simulink model "Stinger"  (R2023a)
settings: Solver=VariableStepAuto  StartTime=0.0  StopTime=20  FixedStep=1e-3  EnableMultiTasking=on
values from neighbouring files (symbols this model uses):
  bp = 0.001    [ControlLawsScript.m]    (also in ControlLaws_Script.m)
  bq = 0.001    [ControlLawsScript.m]    (also in ControlLaws_Script.m)
  br = 0.001    [ControlLawsScript.m]    (also in ControlLaws_Script.m)
  cx = 5    [ControlLawsScript.m]    (also in ControlLaws_Script.m)
  cy = 5    [ControlLawsScript.m]    (also in ControlLaws_Script.m)
  cz = 5    [ControlLawsScript.m]    (also in ControlLaws_Script.m)
  g = 9.80665    [ControlLawsScript.m]    (also in ControlLaws_Script.m; Qball_X8_Model.m = 9.87)
  Kp = (Jx/Tc)-bp    (= 1.02772632451)    [ControlLawsScript.m]    (also in ControlLaws_Script.m = 4.11390529802)
  Kp2 = Jx*((4/ts))*((-4/ts)+((bp+Kp)/Jx))/Kp    (= 1.68163467643)    [ControlLawsScript.m]    (also in ControlLaws_Script.m = 6.72163348437)
  Kq = (Jy/Tc)-bq    (= 1.02971502036)    [ControlLawsScript.m]    (also in ControlLaws_Script.m = 4.12186008142)
  Kq2 = Jy*((4/ts))*((-4/ts)+((bq+Kq)/Jy))/Kq    (= 1.68163151937)    [ControlLawsScript.m]    (also in ControlLaws_Script.m = 6.72163033191)
  Kr = (Jz/Tc)-br    (= 1.98490876719)    [ControlLawsScript.m]    (also in ControlLaws_Script.m = 7.94263506876)
  Kr2 = Jz*((4/ts))*((-4/ts)+((br+Kr)/Jz))/Kr    (= 1.68084638651)    [ControlLawsScript.m]    (also in ControlLaws_Script.m = 6.72084606682)
  kv = 1/930    (= 0.0010752688172)    [StingerScript.m]
  Kx = abs(Kx)    [ControlLawsScript.m]    (also in ControlLaws_Script.m)
  Ky = abs(Ky)    [ControlLawsScript.m]    (also in ControlLaws_Script.m)
  Kz = (m/Tcz)-cz    (= 38.5143536865)    [ControlLawsScript.m]    (also in ControlLaws_Script.m)
  Kz2 = m*((4/tsz))*((-4/tsz)+((cz+Kz)/m))/Kz    (= 1.89810050529)    [ControlLawsScript.m]    (also in ControlLaws_Script.m)
  m = 3.4811482949175    (= 3.48114829492)    [ControlLawsScript.m]    (also in ControlLaws_Script.m; Qball_X8_Model.m = 1.45)
  pitch_angle_limit = pi/6    (= 0.523598775598)    [ControlLawsScript.m]    (also in ControlLaws_Script.m = 0.558505360638)
  R2D = 180/pi    (= 57.2957795131)    [ControlLawsScript.m]    (also in ControlLaws_Script.m)
  roll_angle_limit = pi/6    (= 0.523598775598)    [ControlLawsScript.m]    (also in ControlLaws_Script.m = 0.558505360638)
  z_x = cx    (= 5)    [ControlLawsScript.m]    (also in ControlLaws_Script.m)
  z_y = cy    (= 5)    [ControlLawsScript.m]    (also in ControlLaws_Script.m)
undefined symbols (not defined in the file or in its folder): FC, LAC, LeftAftArm, LeftAftProp, LeftAftSkid, LeftArm, LeftFrontArm, LeftFrontProp, LeftFrontSkid, LeftProp, Lower, missionPlanX, missionPlanY, missionPlanYaw, missionPlanZ, RAC, RightAftArm, RightAftProp, RightAftSkid, RightArm, RightFrontArm, RightFrontProp, RightFrontSkid, RightProp, SC, timeConstant, Upper, X, Y, Z
libraries: sm_lib x98, nesl_utility x56, fl_lib x45, ee_lib x19, batteryecm_lib x2, sharedtransformsys x1, sharedutil x1
(part 1 of 4)
settings Model: Creator=G_MAMAN  LastModifiedBy=alger
settings SolverCC: ZeroCrossAlgorithm=Adaptive  AlgebraicLoopSolver=LineSearch  SolverResetMethod=Robust
settings DataIOCC: LimitDataPoints=on  MaxDataPoints=10000  Refine=5
settings OptimizationCC: LifeSpan=inf
settings DebuggingCC: IgnoredZcDiagnostic=none  UnconnectedInputMsg=warning  UnconnectedOutputMsg=warning  UnconnectedLineMsg=warning  AllowSymbolicDim=off  SFUnexpectedBacktrackingDiag=warning  SFNoUnconditionalDefaultTransitionDiag=warning  SFExecutionAtInitializationDiag=none  ArithmeticOperatorsInVariantConditions=warning
settings ModelReferenceCC: EnableRefExpFcnMdlSchedulingChecks=on
settings SFSimCC: SimUseLocalCustomCode=off  CustomCodeUndefinedFunction=UseInterfaceOnly
settings RTWCC: RTWUseLocalCustomCode=off
settings CodeAppCC: StateflowObjectComments=on
settings GRTTargetCC: TargetLangStandard=C89/C90 (ANSI)
settings ConfigComp: CovMetricSettings=dw  CovSaveCumulativeToWorkspaceVar=on  CovSaveSingleToWorkspaceVar=on  CovExternalEMLEnable=off  CovSFcnEnable=off
settings SimscapeCC: SimscapeLogType=all  SimscapeLogSimulationStatistics=on  SimscapeLogDataHistory=10000
settings DiagnosticsConfigSet: SimMechanicsRigidlyBoundBlock=none
settings ExplorerConfigSet: InternalSimMechanicsExplorerSettings="<ExplorerConfiguration><canonicalview>default</canonicalview><AnimationSetting><BasePlaybackSpeed>1.0</BasePlaybackSpeed><PlaybackSpeedFactor>1.0</PlaybackSpeedFactor></AnimationSetting><TilePanel><TileInfo><Tiles Columns=\"1\" Count=\"1\" Rows=\"1\"><Column Weight=\"1\"/><Row Weight=\"1\"/><Tile Height=\"1\" Width=\"1\" X=\"0\" Y=\"0\"/></Tiles></TileInfo><SceneInfo><SceneViewer><BGColor><R>0</R><G>0</G><B>0</B></BGColor><Camera><DoPerspective>off</DoPerspective><Position><X>7.1395388580893373</X><Y>-9.57545541238177833</Y><Z>5.80767107239631564</Z></Position><Center><X>-0.863567299281931766</X><Y>0.176174380151177173</Y><Z>1.92916926391305155</Z></Center><Up><X>-0.173509302469238902</X><Y>0.237715937307242831</Y><Z>0.955712119367949198</Z></Up><ViewLimDist>1</ViewLimDist><YLim>4.19925208742349287</YLim><XLim>9.96419089960335391</XLim></Camera></SceneViewer></SceneInfo></TilePanel><MechEditorPanel><Cameras/><GfxPanelCameraMap/><VideoCreator><PlaybackSpeedRatio>1.0</PlaybackSpeedRatio><FrameRate>30</FrameRate><VideoFormat>Motion JPEG AVI</VideoFormat><FrameSize>auto</FrameSize></VideoCreator></MechEditorPanel></ExplorerConfiguration>"

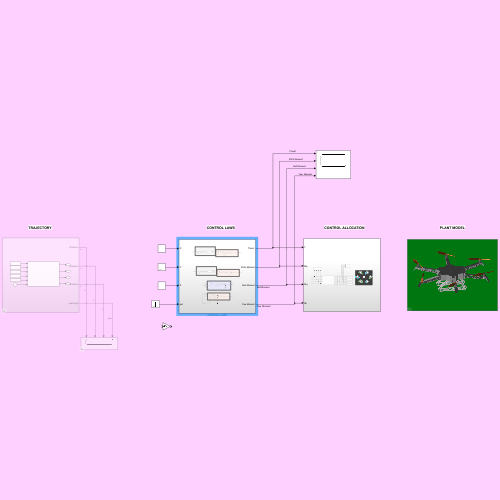
[thumbnail: Simulink's stored preview of the top-level diagram]
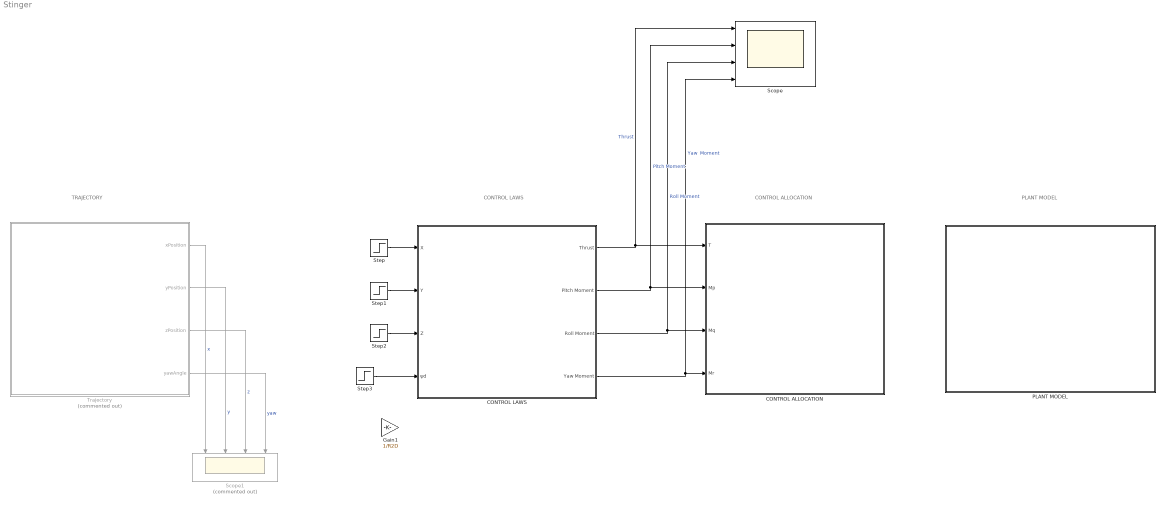
== system Stinger ==
  note: CONTROL LAWS
  note: CONTROL ALLOCATION
  note: PLANT MODEL
  note: TRAJECTORY
  CONTROL ALLOCATION : Subsystem
  CONTROL LAWS : Subsystem
  Gain1 : Gain  Gain=1/R2D
  PLANT MODEL : Subsystem  mask{s=6, g=9.80665, D=0.235, H=0.051, rho=3400, rgb=[0.753 0.753 0.753], op=1}
      mask prompts: s "Shape (# Sides)"; g "Gravitational Acceleration (m/s^2)"; D "Length of Fuselage (m)"; H "Height of Fuselage (m)"; rho "Density of Fuselage (kg/m^3)"; rgb "Color of Fuselage [R G B]"; op "Opacity of Fuselage (0-1)"
      mask Display: image('$imagefile'); % Use "Edit Image" on toolstrip to change.
  Scope : Scope  NumInputPorts=4
  Scope1 : Scope  Commented=on  NumInputPorts=4
  Step : Step  Time=0  After=0  SampleTime=0
  Step1 : Step  Time=0  After=0  SampleTime=0
  Step2 : Step  Time=0  After=4  SampleTime=0
  Step3 : Step  Time=4  After=2  SampleTime=0
  Trajectory : Subsystem  Commented=on
  wires:
  CONTROL LAWS/4(Yaw Moment) -> Scope/4, CONTROL ALLOCATION/4(Mr)  "Yaw  Moment"
  CONTROL LAWS/2(Pitch Moment) -> Scope/2, CONTROL ALLOCATION/2(Mp)  "Pitch Moment"
  CONTROL LAWS/1("Thrust ") -> Scope/1, CONTROL ALLOCATION/1(T)  "Thrust"
  CONTROL LAWS/3(Roll Moment) -> Scope/3, CONTROL ALLOCATION/3(Mq)  "Roll Moment"
  Trajectory/1(xPosition) -> Scope1/1  "x"
  Trajectory/2(yPosition) -> Scope1/2  "y"
  Trajectory/3(zPosition) -> Scope1/3  "z"
  Trajectory/4(yawAngle) -> Scope1/4  "yaw"
  Step/1 -> CONTROL LAWS/1(X)
  Step1/1 -> CONTROL LAWS/2(Y)
  Step2/1 -> CONTROL LAWS/3(Z)
  Step3/1 -> CONTROL LAWS/4(ψd)

== system Stinger/CONTROL ALLOCATION ==
  note: 1
  T : Inport
  Mp : Inport  Port=2
  Mq : Inport  Port=3
  Mr : Inport  Port=4
  Control Allocation : MATLAB Function  TreatAsAtomicUnit=on
  Saturation{6..11} (6 alike) : Saturate  UpperLimit=10000  LowerLimit=0
  Scope : Scope  NumInputPorts=4
  Scope1 : Scope  NumInputPorts=6
  tag scope: ReqSpeedMotor1=global, ReqSpeedMotor2=global, ReqSpeedMotor3=global, ReqSpeedMotor4=global, ReqSpeedMotor5=global, ReqSpeedMotor6=global
  wires:
  T/1 -> Control Allocation/1(T), Scope/1  "T"
  Mp/1 -> Control Allocation/2(Mp), Scope/2  "Mp"
  Mq/1 -> Control Allocation/3(Mq), Scope/3  "Mq"
  Mr/1 -> Control Allocation/4(Mr), Scope/4  "Mr"
  Control Allocation/1(w1) -> Saturation6/1  "1"
  Control Allocation/2(w2) -> Saturation7/1  "2"
  Control Allocation/3(w3) -> Saturation8/1  "3"
  Control Allocation/4(w4) -> Saturation9/1  "4"
  Control Allocation/6(w6) -> Saturation11/1  "6"
  Control Allocation/5(w5) -> Saturation10/1  "5"
  Saturation6/1 -> [ReqSpeedMotor1], Scope1/1
  Saturation10/1 -> Scope1/5, [ReqSpeedMotor5]
  Saturation7/1 -> [ReqSpeedMotor2], Scope1/2
  Saturation9/1 -> Scope1/4, [ReqSpeedMotor4]
  Saturation8/1 -> Scope1/3, [ReqSpeedMotor3]
  Saturation11/1 -> Scope1/6, [ReqSpeedMotor6]

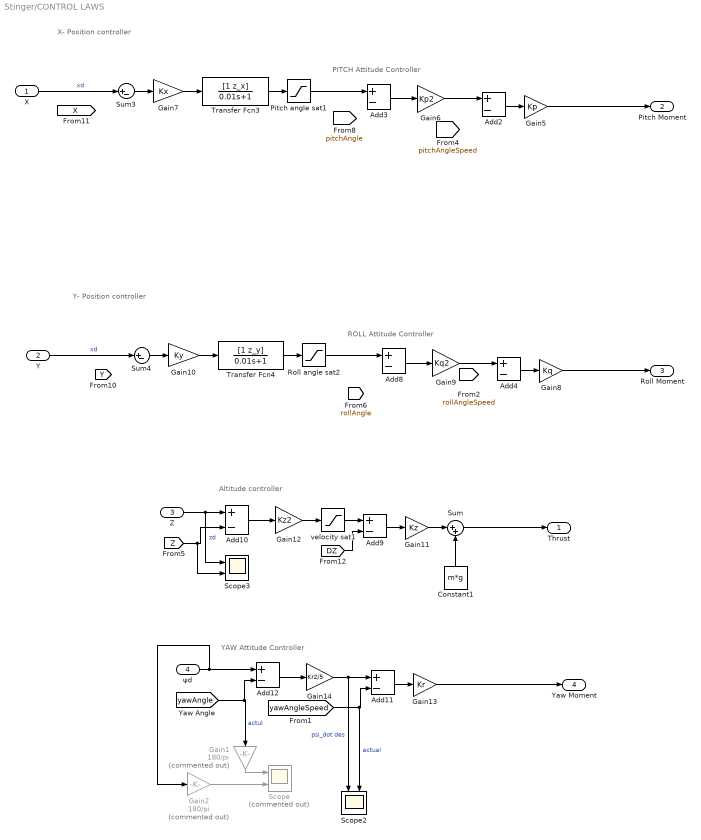
== system Stinger/CONTROL LAWS ==
  note: PITCH Attitude Controller
  note: X- Position controller
  note: YAW Attitude Controller
  note: Y- Position controller
  note: ROLL Attitude Controller
  note: Altitude controller
  X : Inport
  Y : Inport  Port=2
  Z : Inport  Port=3
  ψd : Inport  Port=4
  Add{2..4,8..12} (8 alike) : Sum  Inputs=+-
  Constant1 : Constant  Value=m*g
  Gain1 : Gain  Commented=on  Gain=180/pi
  Gain10 : Gain  Gain=Ky
  Gain11 : Gain  Gain=Kz
  Gain12 : Gain  Gain=Kz2
  Gain13 : Gain  Gain=Kr
  Gain14 : Gain  Gain=Kr2/5
  Gain2 : Gain  Commented=on  Gain=180/pi
  Gain5 : Gain  Gain=Kp
  Gain6 : Gain  Gain=Kp2
  Gain7 : Gain  Gain=Kx
  Gain8 : Gain  Gain=Kq
  Gain9 : Gain  Gain=Kq2
  Pitch angle sat1 : Saturate  UpperLimit=pitch_angle_limit  LowerLimit=-pitch_angle_limit
  Roll angle sat2 : Saturate  UpperLimit=roll_angle_limit  LowerLimit=-roll_angle_limit
  Scope : Scope  Commented=on  NumInputPorts=2
  Scope2 : Scope  NumInputPorts=2
  Scope3 : Scope  NumInputPorts=2
  Sum : Sum  Inputs=|++
  Sum3 : Sum  Inputs=|+-
  Sum4 : Sum  Inputs=|+-
  Transfer Fcn3 : TransferFcn  Numerator=[1 z_x]  Denominator=[0.01 1]
  Transfer Fcn4 : TransferFcn  Numerator=[1 z_y]  Denominator=[0.01 1]
  velocity sat1 : Saturate  UpperLimit=1  LowerLimit=-1
  "Thrust " : Outport
  Pitch Moment : Outport  Port=2
  Roll Moment : Outport  Port=3
  Yaw Moment : Outport  Port=4
  wires:
  Sum4/1 -> Gain10/1
  Gain12/1 -> velocity sat1/1
  Add10/1 -> Gain12/1
  Add9/1 -> Gain11/1
  Add11/1 -> Gain13/1
  [DZ] -> Add9/2
  Transfer Fcn4/1 -> Roll angle sat2/1
  Add4/1 -> Gain8/1
  [Z] -> Scope3/2, Add10/2
  Add12/1 -> Gain14/1
  Gain5/1 -> Pitch Moment/1
  Add2/1 -> Gain5/1
  Y/1 -> Sum4/1  "xd"
  Gain10/1 -> Transfer Fcn4/1
  X/1 -> Sum3/1  "xd"
  Roll angle sat2/1 -> Add8/1
  Sum/1 -> "Thrust "/1
  Constant1/1 -> Sum/2
  Gain9/1 -> Add4/1
  Pitch angle sat1/1 -> Add3/1
  [yawAngleSpeed] -> Add11/2, Scope2/2  "actual"
  Add8/1 -> Gain9/1
  Gain14/1 -> Add11/1, Scope2/1  "psi_dot des"
  Gain6/1 -> Add2/1
  Transfer Fcn3/1 -> Pitch angle sat1/1
  [yawAngle] -> Add12/2, Gain1/1  "actul"
  Add3/1 -> Gain6/1
  Z/1 -> Scope3/1, Add10/1  "zd"
  Gain7/1 -> Transfer Fcn3/1
  Gain8/1 -> Roll Moment/1
  Sum3/1 -> Gain7/1
  Gain11/1 -> Sum/1
  velocity sat1/1 -> Add9/1
  ψd/1 -> Gain2/1, Add12/1
  Gain1/1 -> Scope/1
  Gain13/1 -> Yaw Moment/1
  Gain2/1 -> Scope/2

== system Stinger/PLANT MODEL ==
  BODY : Subsystem  mask{R1=0.025, L1=0.253, theta=0, Rp=0.009}
      mask prompts: R1 "Radius of Arm (m)"; L1 "Length of Arm (m)"; theta "Arm Height Angle (deg)"; Rp "Width of Propeller (m)"
      mask Display: image('$imagefile'); % Use "Edit Image" on toolstrip to change.
  Body : Subsystem
  CONTACT FORCES : Subsystem  mask{st=4e5, b=4e4, trans=1e-4, mus=0.9, mud=0.8, vcr=1e-1}
      mask prompts: st "Stiffness (N/m)"; b "Damping (N/(m/s))"; trans "Transition Region Width (m)"; mus "Coefficient of Static Friction"; mud "Coefficient of Dynamic Friction"; vcr "Critical Velocity (m/s)"
      mask Display: image('$imagefile'); % Use "Edit Image" on toolstrip to change.
  Connection Label : ConnectionLabel  Label=LAC
  Connection Label1 : ConnectionLabel  Label=RAC
  Connection Label2 : ConnectionLabel  Label=SC
  Connection Label3 : ConnectionLabel  Label=MS
  Connection Label4 : ConnectionLabel  Label=MS
  Connection Label5 : ConnectionLabel  Label=LAC
  Connection Label6 : ConnectionLabel  Label=RAC
  Connection Label7 : ConnectionLabel  Label=SC
  Drone Sensors Frame : sm_lib/Frames and Transforms/Reference Frame
  ELECTRIC SYSTEM : Subsystem  mask{F=41.7}
      mask prompts: F "Lift Force (N)"
      mask Display: image('$imagefile'); % Use "Edit Image" on toolstrip to change.
  ENVIRONMENT : Subsystem  mask{E=15, P=0.1, Z=0.12, K=5, BIG=5}
      mask prompts: E "Size of Ground (m)"; P "Height of Ground (m)"; Z "Displacement of Ground (m)"; K "Distance Between Clouds (m)"; BIG "Size of Sun (m)"
      mask Display: image('$imagefile'); % Use "Edit Image" on toolstrip to change.
  Fuselage Contact : ConnectionLabel  Label=FC
  Fuselage Contact1 : ConnectionLabel  Label=FC
  Mechanism Configuration : sm_lib/Utilities/Mechanism Configuration  UniformGravity=Constant  GravityVector=[0 0 -g]  GravityVectorUnits=m/s^2  LinearizationDelta=0.001  JointModeTransitionNonlinearIterations=2
  SENSORS : Subsystem  mask{Parameter1=0}
      mask Display: image('$imagefile'); % Use "Edit Image" on toolstrip to change.
  SKIDS : Subsystem  mask{rho2=788, rgb2=[1 1 1], op2=1}
      mask prompts: rho2 "Density of Skid (kg/m^3)"; rgb2 "Color of Skid [R G B]"; op2 "Opacity of Skid (0-1)"
      mask Display: image('$imagefile'); % Use "Edit Image" on toolstrip to change.
  Simscape Bus : SimscapeBus  HierarchyStrings=FC;LAC;RAC;SC
  Solver Configuration : nesl_utility/Solver Configuration  PhysicalDomain=network_engine_domain  SubClassName=solver  LeftPortType=input  RightPortType=generic  Tones=[]  Harmonics=[]  SimulateNoise=off  Profile=off  UseLocalSampling=off  EnableSwitchedLinearOptims=on  FrequencyDomain=off  UseCCode=off  RelTol=0.001  AbsTol=1e-06  MinStep=1e-09  ToWorkspace=off  RevertToSquareIcSolve=off  NumHomotopyIterations=100  PhasorMode=off  PhasorModeNumHarmonics=1  ConsistencySolver=NEWTON_FTOL  IndexReductionMethod=DerivativeReplacement  DoDC=off  ResidualTolerance=1e-06  ConsistencyTolSource=GLOBAL  ConsistencyAbsTol=0.001  ConsistencyRelTol=0.001  ConsistencyTolFactor=0.001  UseLocalSolver=off  LocalSolverChoice=NE_BACKWARD_EULER_ADVANCER  ResolveIndetEquations=on  FunctionEvalNumThread=1  LocalSolverSampleTime=0.001  DoFixedCost=off  MaxNonlinIter=3  MaxModeIter=2  ComputeImpulses=off  ImpulseIterations=2  LinearAlgebra=auto  LinearAlgebraNumThread=0  EquationFormulation=NE_TIME_EF  DelaysMemoryBudget=1024  AutomaticFiltering=on  FilteringTimeConstant=0.001  PartitionStorageMethod=AS_NEEDED  PartitionMemoryBudget=1024  PartitionMethod=ROBUST
  connections:
  Fuselage Contact/LConn1 -- Body/LConn1
  SKIDS/LConn2 -- BODY/RConn1 -- Connection Label4/LConn1 -- Body/RConn1 -- Solver Configuration/RConn1 -- SENSORS/RConn4 -- Drone Sensors Frame/RConn1 -- Mechanism Configuration/RConn1
  ELECTRIC SYSTEM/LConn1 -- BODY/LConn1
  Connection Label/LConn1 -- BODY/RConn2
  Connection Label1/LConn1 -- BODY/RConn3
  Connection Label2/LConn1 -- SKIDS/LConn1
  Connection Label3/LConn1 -- SENSORS/RConn2
  Fuselage Contact1/LConn1 -- Simscape Bus/LConn1
  Simscape Bus/LConn2 -- Connection Label5/LConn1
  Connection Label6/LConn1 -- Simscape Bus/LConn3
  Simscape Bus/LConn4 -- Connection Label7/LConn1
  Simscape Bus/RConn1 -- CONTACT FORCES/RConn2
  ENVIRONMENT/LConn1 -- CONTACT FORCES/RConn1
  ENVIRONMENT/RConn1 -- SENSORS/RConn3

== system Stinger/Trajectory ==
  Clock : Clock
  Constant : Constant  Value=timeConstant
  Constant1 : Constant  Value=missionPlanX
  Constant2 : Constant  Value=missionPlanY
  Constant3 : Constant  Value=missionPlanZ
  Constant4 : Constant  Value=missionPlanYaw
  Trajectory Control : MATLAB Function  TreatAsAtomicUnit=on
  xPosition : Outport
  yPosition : Outport  Port=2
  zPosition : Outport  Port=3
  yawAngle : Outport  Port=4
  wires:
  Trajectory Control/1(xPosition) -> xPosition/1
  Constant1/1 -> Trajectory Control/1(missionPlanX)
  Constant/1 -> Trajectory Control/5(timeConstant)
  Constant3/1 -> Trajectory Control/3(missionPlanZ)
  Constant2/1 -> Trajectory Control/2(missionPlanY)
  Trajectory Control/3(zPosition) -> zPosition/1
  Trajectory Control/2(yPosition) -> yPosition/1
  Clock/1 -> Trajectory Control/6(simulationTime)
  Constant4/1 -> Trajectory Control/4(missionPlanYaw)
  Trajectory Control/4(yaw) -> yawAngle/1

== system Stinger/PLANT MODEL/BODY ==
  Allocation : Subsystem
  Arms : Subsystem  mask{rho1=1518, rgb1=[0.753 0.753 0.753], op1=1, rhoM=14013}
      mask prompts: rho1 "Density of Arm (kg/m^3)"; rgb1 "Color of Arm [R G B]"; op1 "Opacity of Arm (0-1)"; rhoM "Density of Motors"
      mask Display: image('Arm.jpg'); % Use "Edit Image" on toolstrip to change.
  Propellers : Subsystem  mask{rhoP=2649, rgbP=[1 0.549 0.2], opP=1}
      mask prompts: rhoP "Density of Propeller (kg/m^3)"; rgbP "Color of Propeller [R G B]"; opP "Opacity of Propeller (0-1)"
      mask Display: image('$imagefile'); % Use "Edit Image" on toolstrip to change.
  Fuselage : PMIOPort  Side=Right
  Lift : PMIOPort  Port=2  Side=Left
  Left Contact : PMIOPort  Port=3  Side=Right
  Right Contact : PMIOPort  Port=4  Side=Right
  connections:
  Allocation/RConn1 -- Lift/RConn1
  Propellers/RConn4 -- Allocation/LConn4 -- Arms/LConn4
  Arms/LConn7 -- Fuselage/RConn1
  Arms/RConn1 -- Left Contact/RConn1
  Arms/RConn2 -- Right Contact/RConn1
  Propellers/RConn5 -- Allocation/LConn5 -- Arms/LConn5
  Propellers/RConn6 -- Allocation/LConn6 -- Arms/LConn6
  Propellers/RConn3 -- Allocation/LConn3 -- Arms/LConn3
  Propellers/RConn2 -- Allocation/LConn2 -- Arms/LConn2
  Propellers/RConn1 -- Allocation/LConn1 -- Arms/LConn1

== system Stinger/PLANT MODEL/Body ==
  Lower Body : sm_lib/Body Elements/File Solid  ExtGeomFileName=UAV_VirtualPrototyping\STL files\LowerBody.stl  UnitType=Custom  ExtGeomFileUnits=mm  StepReaderType=HEX  ExportConvexHullGeometry=on  InertiaType=CalculateFromGeometry  Mass=1.038628  MassUnits=kg  CenterOfMass=[0, 0, -1.64462e-2]  CenterOfMassUnits=m  MomentsOfInertia=[5.66226e-3 5.662277e-3 1.11925e-2]  MomentsOfInertiaUnits=kg*m^2  ProductsOfInertia=[0 0 6.64514e-10]  ProductsOfInertiaUnits=kg*m^2  BasedOnType=Density  Density=rho  DensityUnits=kg/m^3  DoExposeReferenceFrame=on  SerializedFrames=<Frames/>  GraphicType=FromGeometry  MarkerShape=Sphere  MarkerSize=10  GraphicVisPropType=SimpleVisualProperties  GraphicDiffuseColor=rgb  GraphicSpecularColor=[0.5 0.5 0.5 1.0]  GraphicAmbientColor=[0.15 0.15 0.15 1.0]  GraphicEmissiveColor=[0.0 0.0 0.0 1.0]  GraphicShininess=75  GraphicOpacity=op
  Simscape Bus : SimscapeBus  HierarchyStrings=Upper;Lower
  Upper Body : sm_lib/Body Elements/File Solid  ExtGeomFileName=UAV_VirtualPrototyping\STL files\UpperBody.stl  UnitType=Custom  ExtGeomFileUnits=mm  StepReaderType=HEX  ExportConvexHullGeometry=on  InertiaType=CalculateFromGeometry  Mass=1.05986327  MassUnits=kg  CenterOfMass=[0 0 1.6454e-2]  CenterOfMassUnits=m  MomentsOfInertia=[5.7148e-3 5.6834e-3 1.12655e-2]  MomentsOfInertiaUnits=kg*m^2  ProductsOfInertia=[0 0 6.7805e-10]  ProductsOfInertiaUnits=kg*m^2  BasedOnType=Density  Density=rho  DensityUnits=kg/m^3  DoExposeReferenceFrame=on  SerializedFrames=<Frames/>  GraphicType=FromGeometry  MarkerShape=Sphere  MarkerSize=10  GraphicVisPropType=SimpleVisualProperties  GraphicDiffuseColor=rgb  GraphicSpecularColor=[0.5 0.5 0.5 1.0]  GraphicAmbientColor=[0.15 0.15 0.15 1.0]  GraphicEmissiveColor=[0.0 0.0 0.0 1.0]  GraphicShininess=75  GraphicOpacity=op
  Contact : PMIOPort  Side=Left
  Plant : PMIOPort  Port=2  Side=Right
  connections:
  Upper Body/LConn1 -- Simscape Bus/LConn1
  Upper Body/RConn1 -- Lower Body/RConn1 -- Plant/RConn1
  Contact/RConn1 -- Simscape Bus/RConn1
  Simscape Bus/LConn2 -- Lower Body/LConn1

== system Stinger/PLANT MODEL/CONTACT FORCES ==
  Left Contact Arms : SimscapeBus  HierarchyStrings=LeftFrontArm;LeftArm;LeftAftArm
  Right Contact Arms : SimscapeBus  HierarchyStrings=RightFrontArm;RightArm;RightAftArm
  Right Contact Skids : SimscapeBus  HierarchyStrings=LeftAftSkid;LeftFrontSkid;RightFrontSkid;RightAftSkid
  Simscape Bus : SimscapeBus  HierarchyStrings=FC;LAC;RAC;SC
  Simscape Bus1 : SimscapeBus  HierarchyStrings=Upper;Lower
  Spatial Contact Force{,1..11} (12 alike) : sm_lib/Forces and Torques/Spatial Contact Force  SenseContactBaseRotation=off  SenseContactBaseTranslation=off  CoefficientOfDynamicFriction=mud  CoefficientOfStaticFriction=mus  NormalDamping=b  NormalDampingUnits=N/(m/s)  SenseContactSignal=off  NormalStiffness=st  NormalStiffnessUnits=N/m  FrictionalCriticalVelocity=vcr  FrictionalCriticalVelocityUnits=m/s  ZeroCrossDetectContactStartAndEnd=off  SenseContactFollowerRotation=off  SenseContactFollowerTranslation=off  FrictionType=SmoothStickSlip  SenseFrictionalForceMagnitude=off  SenseNormalForceMagnitude=off  NormalForceType=SmoothSpringDamper  SenseNormalVelocity=off  SenseSeparationDistance=off  SenseTangentialVelocity=off  NormalTransitionRegionWidth=trans  NormalTransitionRegionWidthUnits=m
  GC : PMIOPort  Side=Right
  PC : PMIOPort  Port=2  Side=Right
  connections:
  Spatial Contact Force/RConn1 -- Spatial Contact Force9/RConn1 -- GC/RConn1 -- Spatial Contact Force5/RConn1 -- Spatial Contact Force7/RConn1 -- Spatial Contact Force8/RConn1 -- Spatial Contact Force10/RConn1 -- Spatial Contact Force11/RConn1 -- Spatial Contact Force6/RConn1 -- Spatial Contact Force4/RConn1 -- Spatial Contact Force3/RConn1 -- Spatial Contact Force2/RConn1 -- Spatial Contact Force1/RConn1
  Right Contact Arms/LConn3 -- Spatial Contact Force6/LConn1
  Right Contact Arms/LConn2 -- Spatial Contact Force5/LConn1
  Right Contact Arms/LConn1 -- Spatial Contact Force4/LConn1
  Left Contact Arms/LConn2 -- Spatial Contact Force2/LConn1
  Spatial Contact Force1/LConn1 -- Left Contact Arms/LConn1
  Left Contact Arms/LConn3 -- Spatial Contact Force3/LConn1
  Right Contact Skids/LConn1 -- Spatial Contact Force11/LConn1
  Right Contact Skids/LConn2 -- Spatial Contact Force10/LConn1
  Spatial Contact Force8/LConn1 -- Right Contact Skids/LConn3
  Right Contact Skids/LConn4 -- Spatial Contact Force7/LConn1
  Simscape Bus/LConn2 -- Left Contact Arms/RConn1
  Simscape Bus/LConn3 -- Right Contact Arms/RConn1
  Simscape Bus/LConn4 -- Right Contact Skids/RConn1
  PC/RConn1 -- Simscape Bus/RConn1
  Simscape Bus1/RConn1 -- Simscape Bus/LConn1
  Spatial Contact Force/LConn1 -- Simscape Bus1/LConn2
  Spatial Contact Force9/LConn1 -- Simscape Bus1/LConn1

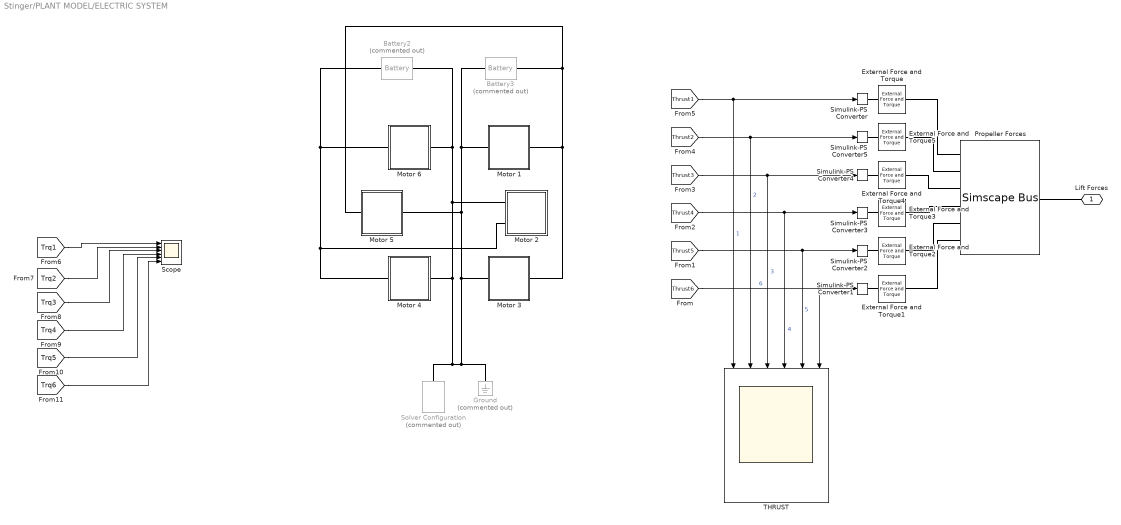
== system Stinger/PLANT MODEL/ELECTRIC SYSTEM ==
  Battery2 : batteryecm_lib/Battery  Commented=on  Vnom=14.8 V  prm_dir=simscape.enum.battery.prm_dir.disabled  R1_dis=2 Ohm  R1_ch=2 Ohm  R1=0.0035*4 Ohm  prm_AH=2  AH=5.2 hr*A  V1=14 V  AH1=2.5 hr*A  prm_R2=1  R2=2000 Ohm  Tmeas=298.15 K  charge_measurement_port=simscape.enum.battery.enable.no  prm_dyn=1  Rp1=0.005 Ohm  tau1=30 s  Rp2=0.005 Ohm  tau2=30 s  Rp3=0.005 Ohm  tau3=30 s  Rp4=0.005 Ohm  tau4=30 s  Rp5=0.005 Ohm  tau5=30 s  prm_fade=1  N_fade=100  AH_fade=45 hr*A  R1_fade=2.02 Ohm  R1_ch_fade=2.02 Ohm  V1_fade=10.35 V  prm_age=simscape.enum.battery.prm_age.disabled  prm_age_OCV=simscape.enum.battery.prm_age_OCV.OCV  OCV_age=0.9  SOC_age=60  Tmeas_age=298.15 K  delta_time_age_vec=[0] d  temperature_age_vec=[273] K  OCV_scaling_age=2.2134e6  OCV_offset_age=1.632e6  temp_exp_age=0.515833569 V  t_exp_age=0.75  Vnom_T2=12 V  R1_T2=2.2 Ohm  R1_T2_dis=2.2 Ohm  R1_T2_ch=2.2 Ohm  V1_T2=11.4 V  R2_T2=2200 Ohm  Rp1_T2=0.005 Ohm  tau1_T2=30 s  Rp2_T2=0.005 Ohm  tau2_T2=30 s  Rp3_T2=0.005 Ohm  tau3_T2=30 s  Rp4_T2=0.005 Ohm  tau4_T2=30 s  Rp5_T2=0.005 Ohm  tau5_T2=30 s  Tmeas2=273.15 K  thermal_port=simscape.enum.thermaleffects.omit  thermal_mass=30000 J/K  i_specify=off  i_priority=None  i=0 A  i_nominal_specify=off  i_nominal_unit=A  i_nominal_value=1  v_specify=off  v_priority=None  v=0 V  v_nominal_specify=off  v_nominal_unit=V  v_nominal_value=1  charge_specify=off  charge_priority=High  charge=50 hr*A  charge_nominal_specify=off  charge_nominal_unit=A*hr  charge_nominal_value=1  num_cycles_specify=off  num_cycles_priority=High  num_cycles=0  num_cycles_nominal_specify=off  num_cycles_nominal_unit=1  num_cycles_nominal_value=1  temperature_specify=off  temperature_priority=High  temperature=298.15 K  temperature_nominal_specify=off  temperature_nominal_unit=K  temperature_nominal_value=1
  Battery3 : batteryecm_lib/Battery  Commented=on  Vnom=14.8 V  prm_dir=simscape.enum.battery.prm_dir.disabled  R1_dis=2 Ohm  R1_ch=2 Ohm  R1=0.0035*4 Ohm  prm_AH=2  AH=5.2 hr*A  V1=14 V  AH1=2.5 hr*A  prm_R2=1  R2=2000 Ohm  Tmeas=298.15 K  charge_measurement_port=simscape.enum.battery.enable.no  prm_dyn=1  Rp1=0.005 Ohm  tau1=30 s  Rp2=0.005 Ohm  tau2=30 s  Rp3=0.005 Ohm  tau3=30 s  Rp4=0.005 Ohm  tau4=30 s  Rp5=0.005 Ohm  tau5=30 s  prm_fade=1  N_fade=100  AH_fade=45 hr*A  R1_fade=2.02 Ohm  R1_ch_fade=2.02 Ohm  V1_fade=10.35 V  prm_age=simscape.enum.battery.prm_age.disabled  prm_age_OCV=simscape.enum.battery.prm_age_OCV.OCV  OCV_age=0.9  SOC_age=60  Tmeas_age=298.15 K  delta_time_age_vec=[0] d  temperature_age_vec=[273] K  OCV_scaling_age=2.2134e6  OCV_offset_age=1.632e6  temp_exp_age=0.515833569 V  t_exp_age=0.75  Vnom_T2=12 V  R1_T2=2.2 Ohm  R1_T2_dis=2.2 Ohm  R1_T2_ch=2.2 Ohm  V1_T2=11.4 V  R2_T2=2200 Ohm  Rp1_T2=0.005 Ohm  tau1_T2=30 s  Rp2_T2=0.005 Ohm  tau2_T2=30 s  Rp3_T2=0.005 Ohm  tau3_T2=30 s  Rp4_T2=0.005 Ohm  tau4_T2=30 s  Rp5_T2=0.005 Ohm  tau5_T2=30 s  Tmeas2=273.15 K  thermal_port=simscape.enum.thermaleffects.omit  thermal_mass=30000 J/K  i_specify=off  i_priority=None  i=0 A  i_nominal_specify=off  i_nominal_unit=A  i_nominal_value=1  v_specify=off  v_priority=None  v=0 V  v_nominal_specify=off  v_nominal_unit=V  v_nominal_value=1  charge_specify=off  charge_priority=High  charge=50 hr*A  charge_nominal_specify=off  charge_nominal_unit=A*hr  charge_nominal_value=1  num_cycles_specify=off  num_cycles_priority=High  num_cycles=0  num_cycles_nominal_specify=off  num_cycles_nominal_unit=1  num_cycles_nominal_value=1  temperature_specify=off  temperature_priority=High  temperature=298.15 K  temperature_nominal_specify=off  temperature_nominal_unit=K  temperature_nominal_value=1
  External Force and Torque{,1..5} (6 alike) : sm_lib/Forces and Torques/External Force and Torque  ForceResolutionFrame=AttachedFrame  EnableForceX=off  EnableForceY=off  EnableForceZ=on  EnableForce=off  TorqueResolutionFrame=AttachedFrame  EnableTorqueX=off  EnableTorqueY=off  EnableTorqueZ=off  EnableTorque=off
  Ground : fl_lib/Electrical/Electrical Elements/Electrical Reference  Commented=on
  Motor 1 : Subsystem
      settings: PortSchema="{\"entries\":[{\"content\":{\"sides\":[{\"content\":{},\"type\":\"ConnectorPlacement.EquallySpacedRectSide\",\"uuid\":\"08d870a7-e796-404b-a5f6-b37f0e33392d\"},{\"content\":{\"side\":\"RIGHT\"},\"type\":\"ConnectorPlacement.EquallySpacedRectSide\",\"uuid\":\"df51a617-9ca1-4f8a-b830-66ef9da37eb2\"},{\"content\":{\"connectorIds\":[\"LConn1\"],\"side\":\"TOP\"},\"type\":\"ConnectorPlacement.EquallySpacedRectSide\",\"uuid\":\"0bf9cc2e-db18-4280-a0b6-874c36a8e80d\"},{\"content\":{\"connectorIds\":[\"RConn1\"],\"side\":\"BOTTOM\"},\"type\":\"ConnectorPlacement.EquallySpacedRectSide\",\"uuid\":\"837a9097-ff08-480d-b5bf-68b48d68c34c\"}]},\"type\":\"ConnectorPlacement.EquallySpacedConnector\",\"uuid\":\"55e23bf7-a9a7-40c2-835c-208173f510f1\"}],\"packageUris\":[\"http://schema.mathworks.com/mf0/Connector/R2020b\"],\"version\":\"1.0\"}"
      mask Display: image('$imagefile'); % Use "Edit Image" on toolstrip to change.
  Motor 2 : Subsystem
      settings: PortSchema="{\"entries\":[{\"content\":{\"sides\":[{\"content\":{},\"type\":\"ConnectorPlacement.EquallySpacedRectSide\",\"uuid\":\"be0e671a-e613-444c-b8e2-6f7a2adfd701\"},{\"content\":{\"side\":\"RIGHT\"},\"type\":\"ConnectorPlacement.EquallySpacedRectSide\",\"uuid\":\"98a92d25-e065-434b-83fd-1db07c9786c9\"},{\"content\":{\"connectorIds\":[\"LConn1\",\"LConn2\"],\"side\":\"TOP\"},\"type\":\"ConnectorPlacement.EquallySpacedRectSide\",\"uuid\":\"6b3cab93-b4c4-4362-9fab-fb0578b34e5e\"},{\"content\":{\"side\":\"BOTTOM\"},\"type\":\"ConnectorPlacement.EquallySpacedRectSide\",\"uuid\":\"096b815e-5cad-442a-9b00-3e24e5e9ca79\"}]},\"type\":\"ConnectorPlacement.EquallySpacedConnector\",\"uuid\":\"7d9f7809-5a51-462b-83e3-36dfed501a9a\"}],\"packageUris\":[\"http://schema.mathworks.com/mf0/Connector/R2020b\"],\"version\":\"1.0\"}"
      mask Display: image('$imagefile'); % Use "Edit Image" on toolstrip to change.
  Motor 3 : Subsystem
      settings: PortSchema="{\"entries\":[{\"content\":{\"sides\":[{\"content\":{},\"type\":\"ConnectorPlacement.EquallySpacedRectSide\",\"uuid\":\"be0e671a-e613-444c-b8e2-6f7a2adfd701\"},{\"content\":{\"side\":\"RIGHT\"},\"type\":\"ConnectorPlacement.EquallySpacedRectSide\",\"uuid\":\"98a92d25-e065-434b-83fd-1db07c9786c9\"},{\"content\":{\"connectorIds\":[\"LConn1\"],\"side\":\"TOP\"},\"type\":\"ConnectorPlacement.EquallySpacedRectSide\",\"uuid\":\"6b3cab93-b4c4-4362-9fab-fb0578b34e5e\"},{\"content\":{\"connectorIds\":[\"RConn1\"],\"side\":\"BOTTOM\"},\"type\":\"ConnectorPlacement.EquallySpacedRectSide\",\"uuid\":\"096b815e-5cad-442a-9b00-3e24e5e9ca79\"}]},\"type\":\"ConnectorPlacement.EquallySpacedConnector\",\"uuid\":\"7d9f7809-5a51-462b-83e3-36dfed501a9a\"}],\"packageUris\":[\"http://schema.mathworks.com/mf0/Connector/R2020b\"],\"version\":\"1.0\"}"
      mask Display: image('$imagefile'); % Use "Edit Image" on toolstrip to change.
  Motor 4 : Subsystem
      settings: PortSchema="{\"entries\":[{\"content\":{\"sides\":[{\"content\":{\"connectorIds\":[]},\"type\":\"ConnectorPlacement.EquallySpacedRectSide\",\"uuid\":\"be0e671a-e613-444c-b8e2-6f7a2adfd701\"},{\"content\":{\"connectorIds\":[],\"side\":\"RIGHT\"},\"type\":\"ConnectorPlacement.EquallySpacedRectSide\",\"uuid\":\"98a92d25-e065-434b-83fd-1db07c9786c9\"},{\"content\":{\"connectorIds\":[\"LConn1\"],\"side\":\"TOP\"},\"type\":\"ConnectorPlacement.EquallySpacedRectSide\",\"uuid\":\"6b3cab93-b4c4-4362-9fab-fb0578b34e5e\"},{\"content\":{\"connectorIds\":[\"RConn1\"],\"side\":\"BOTTOM\"},\"type\":\"ConnectorPlacement.EquallySpacedRectSide\",\"uuid\":\"096b815e-5cad-442a-9b00-3e24e5e9ca79\"}]},\"type\":\"ConnectorPlacement.EquallySpacedConnector\",\"uuid\":\"7d9f7809-5a51-462b-83e3-36dfed501a9a\"}],\"packageUris\":[\"http://schema.mathworks.com/mf0/Connector/19700101\"],\"version\":\"1.0\"}"
      mask Display: image('$imagefile'); % Use "Edit Image" on toolstrip to change.
  Motor 5 : Subsystem
      settings: PortSchema="{\"entries\":[{\"content\":{\"sides\":[{\"content\":{},\"type\":\"ConnectorPlacement.EquallySpacedRectSide\",\"uuid\":\"be0e671a-e613-444c-b8e2-6f7a2adfd701\"},{\"content\":{\"side\":\"RIGHT\"},\"type\":\"ConnectorPlacement.EquallySpacedRectSide\",\"uuid\":\"98a92d25-e065-434b-83fd-1db07c9786c9\"},{\"content\":{\"connectorIds\":[\"LConn1\"],\"side\":\"TOP\"},\"type\":\"ConnectorPlacement.EquallySpacedRectSide\",\"uuid\":\"6b3cab93-b4c4-4362-9fab-fb0578b34e5e\"},{\"content\":{\"connectorIds\":[\"RConn1\"],\"side\":\"BOTTOM\"},\"type\":\"ConnectorPlacement.EquallySpacedRectSide\",\"uuid\":\"096b815e-5cad-442a-9b00-3e24e5e9ca79\"}]},\"type\":\"ConnectorPlacement.EquallySpacedConnector\",\"uuid\":\"7d9f7809-5a51-462b-83e3-36dfed501a9a\"}],\"packageUris\":[\"http://schema.mathworks.com/mf0/Connector/R2020b\"],\"version\":\"1.0\"}"
      mask Display: image('$imagefile'); % Use "Edit Image" on toolstrip to change.
  Motor 6 : Subsystem
      settings: PortSchema="{\"entries\":[{\"content\":{\"sides\":[{\"content\":{},\"type\":\"ConnectorPlacement.EquallySpacedRectSide\",\"uuid\":\"be0e671a-e613-444c-b8e2-6f7a2adfd701\"},{\"content\":{\"side\":\"RIGHT\"},\"type\":\"ConnectorPlacement.EquallySpacedRectSide\",\"uuid\":\"98a92d25-e065-434b-83fd-1db07c9786c9\"},{\"content\":{\"connectorIds\":[\"LConn1\"],\"side\":\"TOP\"},\"type\":\"ConnectorPlacement.EquallySpacedRectSide\",\"uuid\":\"6b3cab93-b4c4-4362-9fab-fb0578b34e5e\"},{\"content\":{\"connectorIds\":[\"RConn1\"],\"side\":\"BOTTOM\"},\"type\":\"ConnectorPlacement.EquallySpacedRectSide\",\"uuid\":\"096b815e-5cad-442a-9b00-3e24e5e9ca79\"}]},\"type\":\"ConnectorPlacement.EquallySpacedConnector\",\"uuid\":\"7d9f7809-5a51-462b-83e3-36dfed501a9a\"}],\"packageUris\":[\"http://schema.mathworks.com/mf0/Connector/R2020b\"],\"version\":\"1.0\"}"
      mask Display: image('$imagefile'); % Use "Edit Image" on toolstrip to change.
  Propeller Forces : SimscapeBus  HierarchyStrings=RightFrontProp;RightProp;RightAftProp;LeftAftProp;LeftProp;LeftFrontProp
  Scope : Scope  NumInputPorts=6
  Simulink-PS Converter{,1..5} (6 alike) : nesl_utility/Simulink-PS Converter  PhysicalDomain=network_engine_domain  SubClassName=ps_input  LeftPortType=input  RightPortType=output  PseudoPeriodic=off  Frequencies=[]  NoiseDistribution=none  NoiseParameters=[]  Unit=N  AffineConversion=off  FilteringAndDerivatives=provide  SimscapeFilterOrder=1  InputFilterTimeConstant=0.001  UdotUserProvided=0
  Solver Configuration : nesl_utility/Solver Configuration  Commented=on  PhysicalDomain=network_engine_domain  SubClassName=solver  LeftPortType=input  RightPortType=generic  Tones=[]  Harmonics=[]  SimulateNoise=off  Profile=off  UseLocalSampling=off  EnableSwitchedLinearOptims=on  FrequencyDomain=off  UseCCode=off  RelTol=0.001  AbsTol=1e-06  MinStep=1e-09  ToWorkspace=off  RevertToSquareIcSolve=off  NumHomotopyIterations=100  PhasorMode=off  PhasorModeNumHarmonics=1  ConsistencySolver=NEWTON_FTOL  IndexReductionMethod=DerivativeReplacement  DoDC=off  ResidualTolerance=1e-06  ConsistencyTolSource=GLOBAL  ConsistencyAbsTol=0.001  ConsistencyRelTol=0.001  ConsistencyTolFactor=0.001  UseLocalSolver=off  LocalSolverChoice=NE_BACKWARD_EULER_ADVANCER  ResolveIndetEquations=on  FunctionEvalNumThread=1  LocalSolverSampleTime=0.001  DoFixedCost=off  MaxNonlinIter=3  MaxModeIter=2  ComputeImpulses=off  ImpulseIterations=2  LinearAlgebra=auto  LinearAlgebraNumThread=0  EquationFormulation=NE_TIME_EF  DelaysMemoryBudget=1024  AutomaticFiltering=on  FilteringTimeConstant=0.001  PartitionStorageMethod=AS_NEEDED  PartitionMemoryBudget=1024  PartitionMethod=ROBUST
  THRUST : Scope  NumInputPorts=6
  Lift Forces : PMIOPort  Side=Left
  wires:
  [Thrust6] -> THRUST/6, Simulink-PS Converter1/1  "6"
  [Thrust5] -> THRUST/5, Simulink-PS Converter2/1  "5"
  [Thrust1] -> Simulink-PS Converter/1, THRUST/1  "1"
  [Thrust2] -> Simulink-PS Converter5/1, THRUST/2  "2"
  [Thrust3] -> THRUST/3, Simulink-PS Converter4/1  "3"
  [Thrust4] -> THRUST/4, Simulink-PS Converter3/1  "4"
  [Trq1] -> Scope/1
  [Trq2] -> Scope/2
  [Trq3] -> Scope/3
  [Trq4] -> Scope/4
  [Trq5] -> Scope/5
  [Trq6] -> Scope/6
  connections:
  Propeller Forces/RConn1 -- Lift Forces/RConn1
  Simulink-PS Converter1/RConn1 -- External Force and Torque1/LConn1
  Simulink-PS Converter2/RConn1 -- External Force and Torque2/LConn1
  Simulink-PS Converter4/RConn1 -- External Force and Torque4/LConn1
  Simulink-PS Converter3/RConn1 -- External Force and Torque3/LConn1
  Simulink-PS Converter5/RConn1 -- External Force and Torque5/LConn1
  External Force and Torque/LConn1 -- Simulink-PS Converter/RConn1
  Motor 4/LConn1 -- Motor 2/LConn2 -- Battery2/LConn1 -- Motor 6/LConn1
  Propeller Forces/LConn1 -- External Force and Torque/RConn1
  External Force and Torque5/RConn1 -- Propeller Forces/LConn2
  Propeller Forces/LConn3 -- External Force and Torque4/RConn1
  Propeller Forces/LConn4 -- External Force and Torque3/RConn1
  Propeller Forces/LConn5 -- External Force and Torque2/RConn1
  Propeller Forces/LConn6 -- External Force and Torque1/RConn1
  Battery3/LConn1 -- Motor 5/LConn1 -- Motor 1/RConn1 -- Motor 3/RConn1
  Motor 5/RConn1 -- Motor 3/LConn1 -- Ground/LConn1 -- Solver Configuration/RConn1 -- Battery2/RConn1 -- Motor 6/RConn1 -- Motor 2/LConn1 -- Motor 4/RConn1 -- Battery3/RConn1 -- Motor 1/LConn1

== system Stinger/PLANT MODEL/ENVIRONMENT ==
  Ground : Subsystem  mask{rhoE=1000000, rgbE=[0 0.7 0.1], opE=1}
      mask prompts: rhoE "Density of Ground (kg/m^3)"; rgbE "Color of Ground [R G B]"; opE "Opacity of Ground (0-1)"
      mask Display: image('ground.jpg'); % Use "Edit Image" on toolstrip to change.
  Sky : Subsystem  mask{rhoS=0.000001, rgbS=[0.529 0.808 0.922], opS=0.5}
      mask prompts: rhoS "Density of Sky (kg/m^3)"; rgbS "Color of Sky [R G B]"; opS "Opacity of Sky (0-1)"
      mask Display: image('sky.jpg'); % Use "Edit Image" on toolstrip to change.
  Tree : Subsystem  mask{rhoB=1000, rgbB=[0.58 0.23 0.19], opB=1}
      mask prompts: rhoB "Density of Buildings (kg/m^3)"; rgbB "Color of Buildings [R G B]"; opB "Opacity of Buildings (0-1)"
      mask Display: image('buildings.jpg'); % Use "Edit Image" on toolstrip to change.
  World Frame : sm_lib/Frames and Transforms/World Frame
  GC : PMIOPort  Side=Left
  World Frame1 : PMIOPort  Port=2  Side=Right
  connections:
  World Frame/RConn1 -- World Frame1/RConn1 -- Ground/RConn1 -- Sky/RConn1 -- Tree/RConn1
  Ground/LConn1 -- GC/RConn1

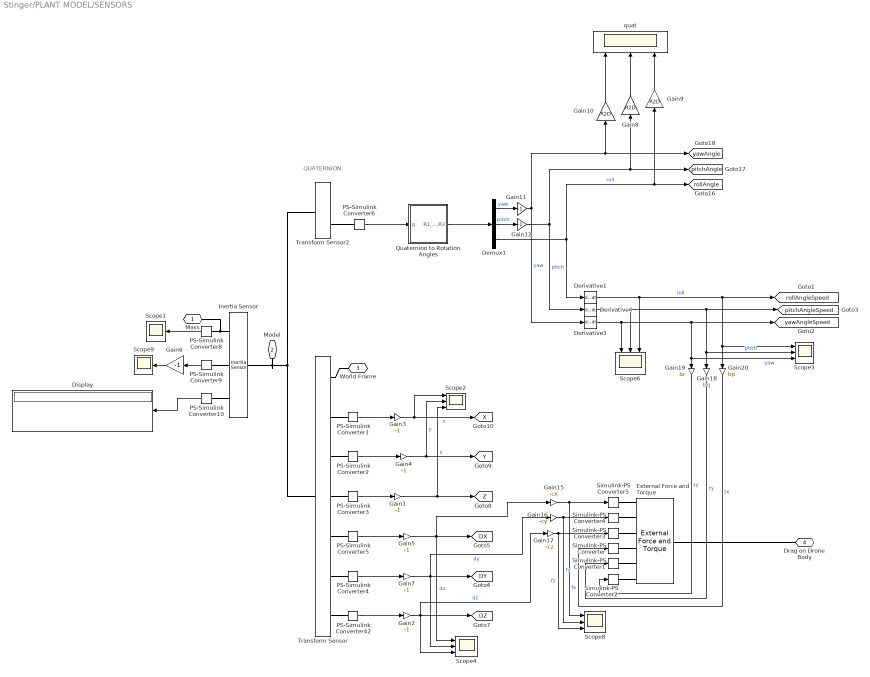
== system Stinger/PLANT MODEL/SENSORS ==
  note: QUATERNION
  Demux1 : Demux  Outputs=3
  Derivative1 : Derivative  CoefficientInTFapproximation=1e-9
  Derivative3 : Derivative  CoefficientInTFapproximation=1e-9
  Derivative4 : Derivative  CoefficientInTFapproximation=1e-9
  Display : Display
  External Force and Torque : sm_lib/Forces and Torques/External Force and Torque  ForceResolutionFrame=AttachedFrame  EnableForceX=on  EnableForceY=on  EnableForceZ=on  EnableForce=off  TorqueResolutionFrame=AttachedFrame  EnableTorqueX=on  EnableTorqueY=on  EnableTorqueZ=on  EnableTorque=off
  Gain{1..7,11..12} (9 alike) : Gain  Gain=-1
  Gain10 : Gain  Gain=R2D
  Gain15 : Gain  Gain=-cx
  Gain16 : Gain  Gain=-cy
  Gain17 : Gain  Gain=-cz
  Gain18 : Gain  Gain=bq
  Gain19 : Gain  Gain=br
  Gain20 : Gain  Gain=bp
  Gain8 : Gain  Gain=R2D
  Gain9 : Gain  Gain=R2D
  Inertia Sensor : sm_lib/Body Elements/Inertia Sensor  SensorExtent=BodyGroup  SpanWeldJoints=off  ExcludeGroundedBodies=off  MeasurementFrame=Attached  SenseMass=on  SenseCenterOfMass=on  SenseInertiaMatrix=on  SenseCenteredInertiaMatrix=off  SensePrincipalInertiaMatrix=off  SenseRotationMatrix=off  GraphicType=None  PrincipalInertiaFrameSize=20  GraphicVisPropType=SimpleVisualProperties  GraphicDiffuseColor=[0.5 0.5 0.5]  GraphicSpecularColor=[0.5 0.5 0.5 1.0]  GraphicAmbientColor=[0.15 0.15 0.15 1.0]  GraphicEmissiveColor=[0.0 0.0 0.0 1.0]  GraphicShininess=75  GraphicOpacity=1.0
  PS-Simulink Converter{1..6,8..9,42} (9 alike) : nesl_utility/PS-Simulink Converter  PhysicalDomain=network_engine_domain  SubClassName=ps_output  LeftPortType=input  RightPortType=output  PseudoPeriodic=off  Frequencies=[]  VectorFormat=1-D array  Unit=inherit  AffineConversion=off
  PS-Simulink Converter10 : nesl_utility/PS-Simulink Converter  PhysicalDomain=network_engine_domain  SubClassName=ps_output  LeftPortType=input  RightPortType=output  PseudoPeriodic=off  Frequencies=[]  VectorFormat=inherit  Unit=inherit  AffineConversion=on
  Quaternion to Rotation Angles : Subsystem
  Scope1 : Scope
  Scope{2..4,6,8} (5 alike) : Scope  NumInputPorts=3
  Scope9 : Scope
  Simulink-PS Converter{,1..5} (6 alike) : nesl_utility/Simulink-PS Converter  PhysicalDomain=network_engine_domain  SubClassName=ps_input  LeftPortType=input  RightPortType=output  PseudoPeriodic=off  Frequencies=[]  NoiseDistribution=none  NoiseParameters=[]  Unit=1  AffineConversion=off  FilteringAndDerivatives=provide  SimscapeFilterOrder=1  InputFilterTimeConstant=0.001  UdotUserProvided=0
  Transform Sensor : sm_lib/Frames and Transforms/Transform Sensor  MeasurementFrame=World  RotationSequence=ZYX  SenseAngle=off  SenseAxis=off  SenseQ=off  SenseR=off  SenseRotationSequence=off  SenseOmegaX=off  SenseOmegaY=off  SenseOmegaZ=off  SenseQDot=off  SenseRDot=off  SenseRotationSequenceDot=off  SenseAlphaX=off  SenseAlphaY=off  SenseAlphaZ=off  SenseQDDot=off  SenseRDDot=off  SenseX=on  SenseY=on  SenseZ=on  SenseRad=off  SenseAzim=off  SenseDist=off  SenseInc=off  SenseXDot=on  SenseYDot=on  SenseZDot=on  SenseRadDot=off  SenseAzimDot=off  SenseDistDot=off  SenseIncDot=off  SenseXDDot=off  SenseYDDot=off  SenseZDDot=off  SenseRadDDot=off  SenseAzimDDot=off  SenseDistDDot=off  SenseIncDDot=off
  Transform Sensor2 : sm_lib/Frames and Transforms/Transform Sensor  MeasurementFrame=World  RotationSequence=ZYX  SenseAngle=off  SenseAxis=off  SenseQ=on  SenseR=off  SenseRotationSequence=off  SenseOmegaX=off  SenseOmegaY=off  SenseOmegaZ=off  SenseQDot=off  SenseRDot=off  SenseRotationSequenceDot=off  SenseAlphaX=off  SenseAlphaY=off  SenseAlphaZ=off  SenseQDDot=off  SenseRDDot=off  SenseX=off  SenseY=off  SenseZ=off  SenseRad=off  SenseAzim=off  SenseDist=off  SenseInc=off  SenseXDot=off  SenseYDot=off  SenseZDot=off  SenseRadDot=off  SenseAzimDot=off  SenseDistDot=off  SenseIncDot=off  SenseXDDot=off  SenseYDDot=off  SenseZDDot=off  SenseRadDDot=off  SenseAzimDDot=off  SenseDistDDot=off  SenseIncDDot=off
  quat : Scope  NumInputPorts=3
  Mass : PMIOPort  Side=Right
  Model : PMIOPort  Port=2  Side=Right
  World Frame : PMIOPort  Port=3  Side=Right
  Drag on Drone Body : PMIOPort  Port=4  Side=Right
  tag scope: DX=global, DY=global, DZ=global, X=global, Y=global, Z=global, pitchAngle=global, pitchAngleSpeed=global, rollAngle=global, rollAngleSpeed=global, yawAngle=global, yawAngleSpeed=global
  wires:
  PS-Simulink Converter9/1 -> Gain6/1
  Gain6/1 -> Scope9/1
  PS-Simulink Converter8/1 -> Scope1/1
  PS-Simulink Converter42/1 -> Gain2/1
  PS-Simulink Converter1/1 -> Gain3/1
  PS-Simulink Converter3/1 -> Gain1/1
  PS-Simulink Converter2/1 -> Gain4/1
  Gain2/1 -> Scope4/3, Gain17/1, [DZ]  "dz"
  Gain1/1 -> Scope2/3, [Z]  "z"
  PS-Simulink Converter4/1 -> Gain7/1
  PS-Simulink Converter5/1 -> Gain5/1
  Gain3/1 -> Scope2/1, [X]  "x"
  Gain4/1 -> [Y], Scope2/2  "y"
  Gain5/1 -> Gain15/1, [DX], Scope4/1  "dx"
  Gain7/1 -> [DY], Gain16/1, Scope4/2  "dy"
  Gain12/1 -> [pitchAngle], Gain8/1, Derivative4/1  "pitch"
  Demux1/3 -> [rollAngle], Gain9/1, Derivative1/1  "roll"
  Demux1/2 -> Gain12/1  "pitch"
  Demux1/1 -> Gain11/1  "yaw"
  Quaternion to Rotation Angles/1(R1,R2,R3) -> Demux1/1
  PS-Simulink Converter6/1 -> Quaternion to Rotation Angles/1(q)
  Gain15/1 -> Scope8/1, Simulink-PS Converter5/1  "fx"
  Gain16/1 -> Scope8/2, Simulink-PS Converter4/1  "fy"
  Gain17/1 -> Scope8/3, Simulink-PS Converter3/1  "fz"
  Gain10/1 -> quat/1
  Gain8/1 -> quat/2
  Gain9/1 -> quat/3
  Derivative3/1 -> Scope3/3, Gain19/1, [yawAngleSpeed], Scope6/1  "yaw"
  Derivative4/1 -> Scope3/2, Gain18/1, [pitchAngleSpeed], Scope6/2  "pitch"
  Derivative1/1 -> [rollAngleSpeed], Scope3/1, Gain20/1, Scope6/3  "roll"
  Gain19/1 -> Simulink-PS Converter2/1  "tz"
  Gain18/1 -> Simulink-PS Converter1/1  "ty"
  Gain20/1 -> Simulink-PS Converter/1  "tx"
  Gain11/1 -> Derivative3/1, [yawAngle], Gain10/1  "yaw"
  PS-Simulink Converter10/1 -> Display/1
  connections:
  PS-Simulink Converter8/LConn1 -- Mass/RConn1 -- Inertia Sensor/RConn1
  PS-Simulink Converter9/LConn1 -- Inertia Sensor/RConn2
  PS-Simulink Converter10/LConn1 -- Inertia Sensor/RConn3
  Model/RConn1 -- Transform Sensor2/LConn1 -- Transform Sensor/LConn1 -- Inertia Sensor/LConn1
  Drag on Drone Body/RConn1 -- External Force and Torque/RConn1
  Simulink-PS Converter/RConn1 -- External Force and Torque/LConn4
  Simulink-PS Converter1/RConn1 -- External Force and Torque/LConn5
  Simulink-PS Converter2/RConn1 -- External Force and Torque/LConn6
  Simulink-PS Converter3/RConn1 -- External Force and Torque/LConn3
  Simulink-PS Converter4/RConn1 -- External Force and Torque/LConn2
  Simulink-PS Converter5/RConn1 -- External Force and Torque/LConn1
  World Frame/RConn1 -- Transform Sensor/RConn1
  PS-Simulink Converter6/LConn1 -- Transform Sensor2/RConn2
  PS-Simulink Converter1/LConn1 -- Transform Sensor/RConn2
  PS-Simulink Converter3/LConn1 -- Transform Sensor/RConn4
  PS-Simulink Converter2/LConn1 -- Transform Sensor/RConn3
  PS-Simulink Converter5/LConn1 -- Transform Sensor/RConn5
  PS-Simulink Converter4/LConn1 -- Transform Sensor/RConn6
  PS-Simulink Converter42/LConn1 -- Transform Sensor/RConn7
